simulink model "nonlinear_vs_linear"  (R2023a)
settings: Solver=ode1  StartTime=0.0  StopTime=200  FixedStep=1e-4  RelTol=1e-3
values from neighbouring files (symbols this model uses):
  alpha = 5    [comparison_of_two_C3s_for_positivity_issue.m]    (also in error_plots.m = 80; ns_vs_ls_sim.m = 80; output_response_gap_metrc_is_1.m = 80)
  beta = params(5)    [NS_parameter_generation.m]    (also in NS_parameter_generation_v2.m = params(4); comparison_of_two_C3s_for_positivity_issue.m = 75; error_plots.m = 75; ns_vs_ls_sim.m = 75)
  e3_0 = 2*(xr0 - x0(4))    [comparison_of_two_C3s_for_positivity_issue.m]    (also in error_plots.m; ns_vs_ls_sim.m; output_response_gap_metrc_is_1.m)
  eta = 75    [comparison_of_two_C3s_for_positivity_issue.m]    (also in error_plots.m; ns_vs_ls_sim.m; output_response_gap_metrc_is_1.m)
  K = 0.12    [comparison_of_two_C3s_for_positivity_issue.m]    (also in error_plots.m; ns_vs_ls_sim.m; output_response_gap_metrc_is_1.m)
  Ks = 0.15    [comparison_of_two_C3s_for_positivity_issue.m]    (also in error_plots.m; ns_vs_ls_sim.m; output_response_gap_metrc_is_1.m)
  Lambda = .08    (= 0.08)    [comparison_of_two_C3s_for_positivity_issue.m]    (also in error_plots.m; ns_vs_ls_sim.m; output_response_gap_metrc_is_1.m)
  x0 = [0;1e-8;0;500e-9]    [comparison_of_two_C3s_for_positivity_issue.m]    (also in error_plots.m; ns_vs_ls_sim.m = [5e-9;0e-5;0;500e-9]; output_response_gap_metrc_is_1.m = [5e-9;0;0;500e-9])
settings Model: Creator=guanyunliu  LastModifiedBy=guanyunliu

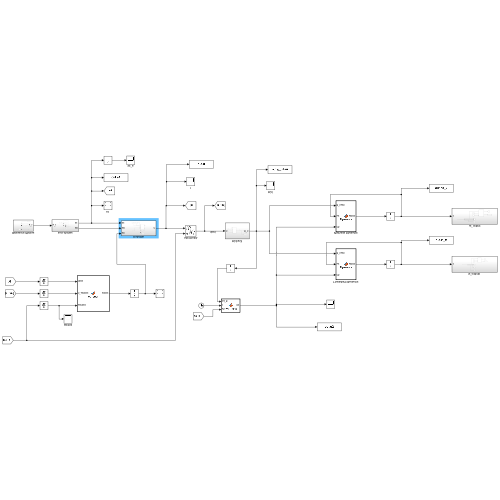
[thumbnail: Simulink's stored preview of the top-level diagram]
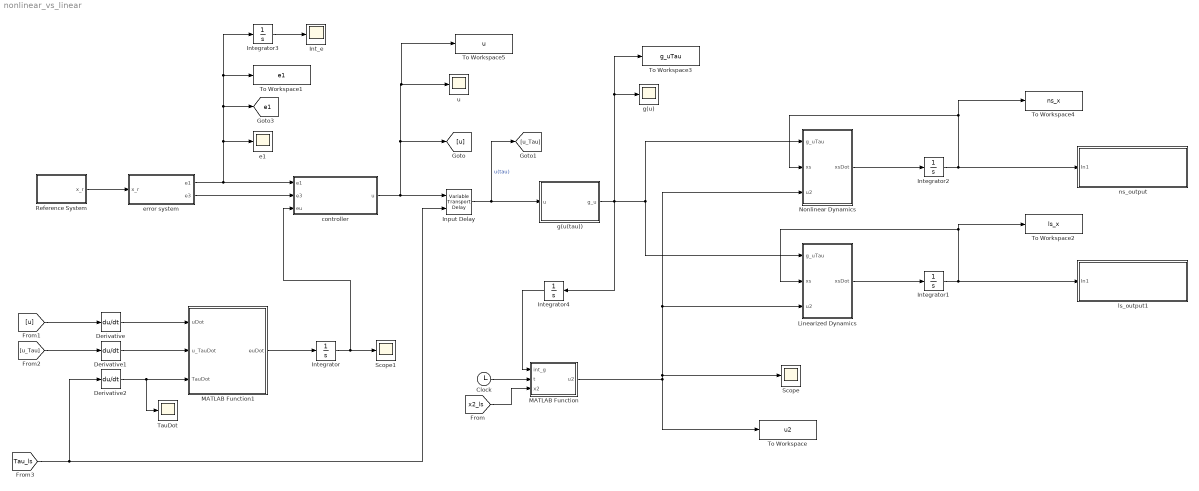
== system nonlinear_vs_linear ==
  Clock : Clock
  Derivative : Derivative
  Derivative1 : Derivative
  Derivative2 : Derivative
  Input Delay : VariableTransportDelay  VariableDelayType=Variable transport delay  MaximumDelay=10  MaximumPoints=100352
  Int_e : Scope
  Integrator : Integrator
  Integrator1 : Integrator  InitialCondition=x0
  Integrator2 : Integrator  InitialCondition=x0
  Integrator3 : Integrator
  Integrator4 : Integrator
  Linearized Dynamics : MATLAB Function  TreatAsAtomicUnit=on
  MATLAB Function : MATLAB Function  TreatAsAtomicUnit=on
  MATLAB Function1 : MATLAB Function  TreatAsAtomicUnit=on
  Nonlinear Dynamics : MATLAB Function  TreatAsAtomicUnit=on
  Reference System : Subsystem
  Scope : Scope
  Scope1 : Scope
  TauDot : Scope
  To Workspace : ToWorkspace  VariableName=u2  SaveFormat=Timeseries  SampleTime=-1
  To Workspace1 : ToWorkspace  VariableName=e1  SaveFormat=Timeseries  SampleTime=-1
  To Workspace2 : ToWorkspace  VariableName=ls_x  SaveFormat=Timeseries  SampleTime=-1
  To Workspace3 : ToWorkspace  VariableName=g_uTau  SaveFormat=Timeseries  SampleTime=-1
  To Workspace4 : ToWorkspace  VariableName=ns_x  SaveFormat=Timeseries  SampleTime=-1
  To Workspace5 : ToWorkspace  VariableName=u  SaveFormat=Timeseries  SampleTime=-1
  controller : Subsystem
  e1 : Scope
  error system : Subsystem
  g(u(tau)) : Subsystem
  g(u) : Scope
  ls_output1 : Subsystem
  ns_output : Subsystem
  u : Scope
  tag scope: e1=global
  wires:
  Reference System/1(x_r) -> error system/1(x_r)
  error system/1(e1) -> controller/1(e1), [e1], Integrator3/1, To Workspace1/1, e1/1
  error system/2(e3) -> controller/2(e3)
  controller/1(u) -> To Workspace5/1, u/1, [u], Input Delay/1
  Input Delay/1 -> [u_Tau], g(u(tau))/1(u)  "u(tau)"
  g(u(tau))/1(g_u) -> Integrator4/1, To Workspace3/1, g(u)/1, Nonlinear Dynamics/1(g_uTau), Linearized Dynamics/1(g_uTau)
  Nonlinear Dynamics/1(xsDot) -> Integrator2/1
  Linearized Dynamics/1(xsDot) -> Integrator1/1
  Integrator2/1 -> To Workspace4/1, Nonlinear Dynamics/2(xs), ns_output/1(In1)
  Integrator1/1 -> To Workspace2/1, Linearized Dynamics/2(xs), ls_output1/1(In1)
  [u_Tau] -> Derivative1/1
  MATLAB Function1/1(euDot) -> Integrator/1
  [u] -> Derivative/1
  Derivative/1 -> MATLAB Function1/1(uDot)
  Derivative1/1 -> MATLAB Function1/2(u_TauDot)
  Derivative2/1 -> TauDot/1, MATLAB Function1/3(TauDot)
  Integrator/1 -> Scope1/1, controller/3(eu)
  [Tau_ls] -> Derivative2/1, Input Delay/2
  MATLAB Function/1(u2) -> Scope/1, Nonlinear Dynamics/3(u2), Linearized Dynamics/3(u2), To Workspace/1
  Integrator3/1 -> Int_e/1
  Clock/1 -> MATLAB Function/2(t)
  Integrator4/1 -> MATLAB Function/1(int_g)
  [x2_ls] -> MATLAB Function/3(x2)

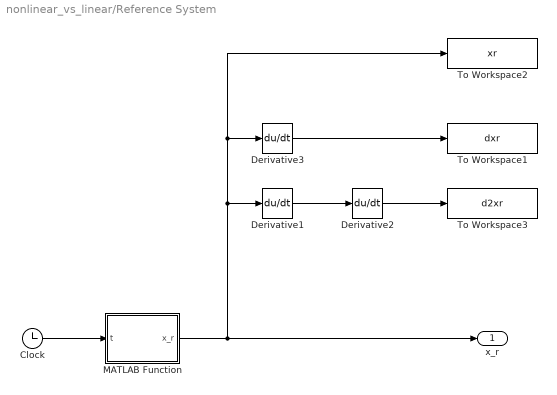
== system nonlinear_vs_linear/Reference System ==
  Clock : Clock
  Derivative1 : Derivative
  Derivative2 : Derivative
  Derivative3 : Derivative
  MATLAB Function : MATLAB Function  TreatAsAtomicUnit=on
  To Workspace1 : ToWorkspace  VariableName=dxr  SaveFormat=Timeseries  SampleTime=-1
  To Workspace2 : ToWorkspace  VariableName=xr  SaveFormat=Timeseries  SampleTime=-1
  To Workspace3 : ToWorkspace  VariableName=d2xr  SaveFormat=Timeseries  SampleTime=-1
  x_r : Outport
  wires:
  Clock/1 -> MATLAB Function/1(t)
  MATLAB Function/1(x_r) -> To Workspace2/1, Derivative3/1, Derivative1/1, x_r/1
  Derivative1/1 -> Derivative2/1
  Derivative2/1 -> To Workspace3/1
  Derivative3/1 -> To Workspace1/1

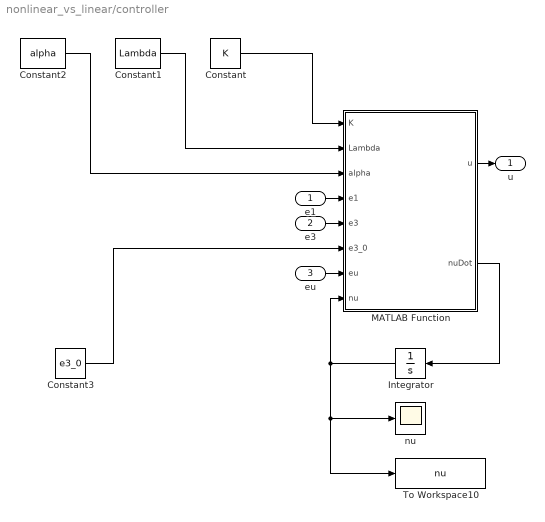
== system nonlinear_vs_linear/controller ==
  e1 : Inport
  e3 : Inport  Port=2
  eu : Inport  Port=3
  Constant : Constant  Value=K
  Constant1 : Constant  Value=Lambda
  Constant2 : Constant  Value=alpha
  Constant3 : Constant  Value=e3_0
  Integrator : Integrator
  MATLAB Function : MATLAB Function  TreatAsAtomicUnit=on
  To Workspace10 : ToWorkspace  VariableName=nu  SaveFormat=Timeseries  SampleTime=-1
  nu : Scope
  u : Outport
  wires:
  MATLAB Function/1(u) -> u/1
  e3/1 -> MATLAB Function/5(e3)
  Constant2/1 -> MATLAB Function/3(alpha)
  Constant/1 -> MATLAB Function/1(K)
  Constant3/1 -> MATLAB Function/6(e3_0)
  Constant1/1 -> MATLAB Function/2(Lambda)
  MATLAB Function/2(nuDot) -> Integrator/1
  e1/1 -> MATLAB Function/4(e1)
  Integrator/1 -> nu/1, To Workspace10/1, MATLAB Function/8(nu)
  eu/1 -> MATLAB Function/7(eu)

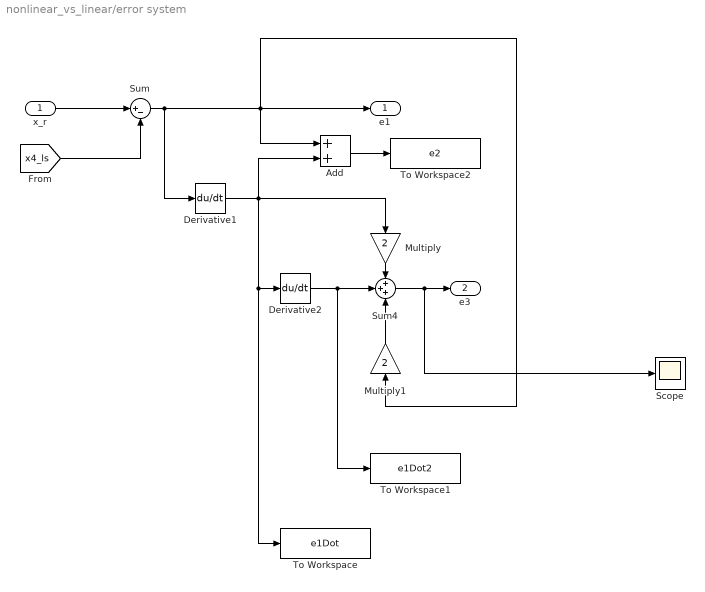
== system nonlinear_vs_linear/error system ==
  x_r : Inport
  Add : Sum
  Derivative1 : Derivative
  Derivative2 : Derivative
  Multiply : Gain  Gain=2
  Multiply1 : Gain  Gain=2
  Scope : Scope
  Sum : Sum  Inputs=|+-
  Sum4 : Sum  Inputs=+++
  To Workspace : ToWorkspace  VariableName=e1Dot  SaveFormat=Timeseries  SampleTime=-1
  To Workspace1 : ToWorkspace  VariableName=e1Dot2  SaveFormat=Timeseries  SampleTime=-1
  To Workspace2 : ToWorkspace  VariableName=e2  SaveFormat=Timeseries  SampleTime=-1
  e1 : Outport
  e3 : Outport  Port=2
  wires:
  x_r/1 -> Sum/1
  [x4_ls] -> Sum/2
  Sum/1 -> Derivative1/1, Add/1, e1/1, Multiply1/1
  Derivative2/1 -> To Workspace1/1, Sum4/2
  Multiply/1 -> Sum4/1
  Multiply1/1 -> Sum4/3
  Sum4/1 -> Scope/1, e3/1
  Derivative1/1 -> Add/2, Multiply/1, To Workspace/1, Derivative2/1
  Add/1 -> To Workspace2/1

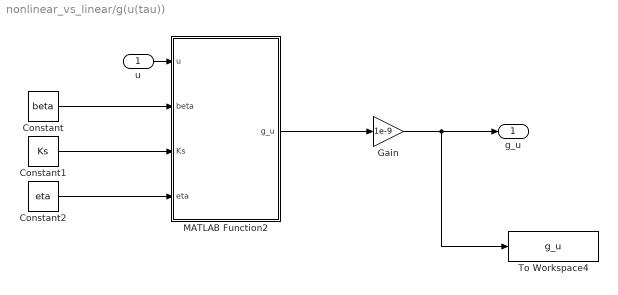
== system nonlinear_vs_linear/g(u(tau)) ==
  u : Inport
  Constant : Constant  Value=beta
  Constant1 : Constant  Value=Ks
  Constant2 : Constant  Value=eta
  Gain : Gain  Gain=1e-9
  MATLAB Function2 : MATLAB Function  TreatAsAtomicUnit=on
  To Workspace4 : ToWorkspace  VariableName=g_u  SaveFormat=Timeseries  SampleTime=-1
  g_u : Outport
  wires:
  Constant1/1 -> MATLAB Function2/3(Ks)
  Constant/1 -> MATLAB Function2/2(beta)
  u/1 -> MATLAB Function2/1(u)
  MATLAB Function2/1(g_u) -> Gain/1
  Constant2/1 -> MATLAB Function2/4(eta)
  Gain/1 -> To Workspace4/1, g_u/1

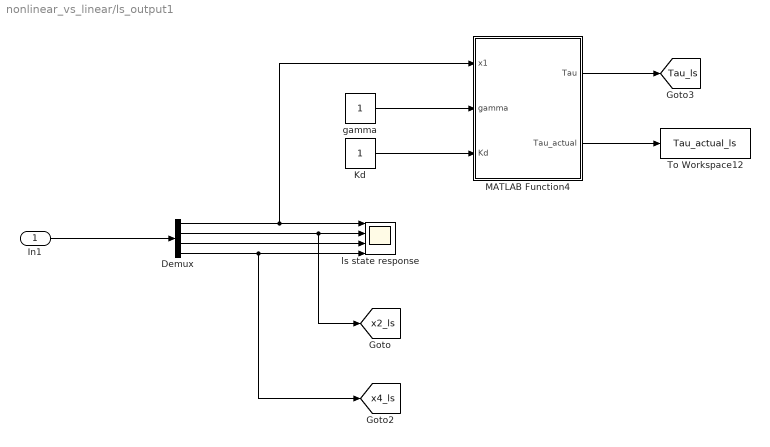
== system nonlinear_vs_linear/ls_output1 ==
  In1 : Inport
  Demux : Demux
  Kd : Constant
  MATLAB Function4 : MATLAB Function  TreatAsAtomicUnit=on
  To Workspace12 : ToWorkspace  VariableName=Tau_actual_ls  SaveFormat=Timeseries  SampleTime=-1
  gamma : Constant
  ls state response : Scope  NumInputPorts=4
  tag scope: Tau_ls=global, x2_ls=global, x4_ls=global
  wires:
  In1/1 -> Demux/1
  MATLAB Function4/2(Tau_actual) -> To Workspace12/1
  MATLAB Function4/1(Tau) -> [Tau_ls]
  Demux/1 -> MATLAB Function4/1(x1), ls state response/1
  Demux/4 -> [x4_ls], ls state response/4
  Kd/1 -> MATLAB Function4/3(Kd)
  gamma/1 -> MATLAB Function4/2(gamma)
  Demux/2 -> [x2_ls], ls state response/2
  Demux/3 -> ls state response/3

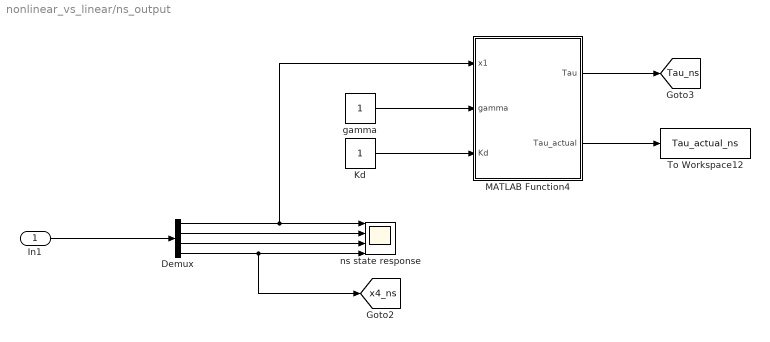
== system nonlinear_vs_linear/ns_output ==
  In1 : Inport
  Demux : Demux
  Kd : Constant
  MATLAB Function4 : MATLAB Function  TreatAsAtomicUnit=on
  To Workspace12 : ToWorkspace  VariableName=Tau_actual_ns  SaveFormat=Timeseries  SampleTime=-1
  gamma : Constant
  ns state response : Scope  NumInputPorts=4
  tag scope: Tau_ns=global, x4_ns=global
  wires:
  In1/1 -> Demux/1
  MATLAB Function4/2(Tau_actual) -> To Workspace12/1
  MATLAB Function4/1(Tau) -> [Tau_ns]
  Demux/1 -> MATLAB Function4/1(x1), ns state response/1
  Demux/4 -> [x4_ns], ns state response/4
  Kd/1 -> MATLAB Function4/3(Kd)
  gamma/1 -> MATLAB Function4/2(gamma)
  Demux/2 -> ns state response/2
  Demux/3 -> ns state response/3

== matlab function nonlinear_vs_linear/controller/MATLAB Function ==
  data: K input; u output; Lambda input; alpha input; e1 input; e3 input; e3_0 input; eu input; nu input; nuDot output
function [u, nuDot] = controller_u(K, Lambda, alpha, e1, e3, e3_0, eu, nu)
u = (sign(0.5 * (sign(e1) + 1))) * ...
    (K * (e3 - e3_0) + nu);
% if u <=0
%     u = 0;
% end
nuDot = K * (Lambda*e3+alpha*eu);
return

== matlab function nonlinear_vs_linear/Linearized Dynamics ==
  data: g_uTau input; xsDot output; xs input; u2 input; params parameter
function xsDot = Dynamics(g_uTau, xs, u2, params)
% xsDot = linearize_ode(xs, g_uTau, params);
xsDot = linearize_ode(xs, g_uTau, u2, params);

== matlab function nonlinear_vs_linear/g(u(tau))/MATLAB Function2 ==
  data: u input; g_u output; beta input; Ks input; eta input
function g_u = controller_g(u,beta, Ks, eta)

% g_u = ((beta/2)+((beta/2)*tanh(Ks/2*(u*1e9 - eta))))*1e-9;
g_u = ((beta/2)+((beta/2)*tanh(Ks/2*(u*1e9 - eta))));

return

== matlab function nonlinear_vs_linear/Nonlinear Dynamics ==
  data: g_uTau input; xsDot output; xs input; u2 input; params parameter
function xsDot = Dynamics(g_uTau, xs, u2, params)
% xsDot = nonlinear_ode(xs, g_uTau, params);
xsDot = nonlinear_ode(xs, g_uTau, u2, params);

== matlab function nonlinear_vs_linear/ns_output/MATLAB Function4 ==
  data: x1 input; Tau output; gamma input; Kd input; Tau_actual output
function [Tau, Tau_actual]= Delay(x1, gamma, Kd)
% Tau=(4.48*(max(x3,.202)^(-0.323))) ; From Damon's code
% Tau = gamma * x3^(-Kd);
Tau = gamma * 5^(-Kd);
Tau_actual = gamma * x1^(-Kd);
return

== matlab function nonlinear_vs_linear/ls_output1/MATLAB Function4 ==
  data: x1 input; Tau output; gamma input; Kd input; Tau_actual output
function [Tau, Tau_actual]= Delay(x1, gamma, Kd)
% Tau=(4.48*(max(x3,.202)^(-0.323))) ; From Damon's code
% Tau = gamma * x3^(-Kd);
% Tau = gamma * 5^(-Kd);
Tau = 0.2;
% Tau = 5;
if x1*1e3 <=0.1e-9
    Tau_actual = 10;
else 
    Tau_actual = gamma * (x1*1e3*1e9)^(-Kd);
end
% Tau = Tau_actual;
return

== matlab function nonlinear_vs_linear/MATLAB Function1 ==
  data: uDot input; euDot output; u_TauDot input; TauDot input
function euDot = eu_error(uDot,u_TauDot, TauDot)

euDot = -uDot+(1-TauDot)*u_TauDot;

== matlab function nonlinear_vs_linear/MATLAB Function ==
  data: int_g input; t input; x2 input; u2 output; params parameter
function u2 = FVII_Input(int_g, t, x2, params)
% u2 is calculated based on the magnitude of the ref signal at the steady
% state

% Regulation
% xr_ss = 130e-9;

% Sinusoidal Tracking
xr_ss = ref_signal(t);

% u2_trans = (-tanh(.2*t-2)+1)*0.5*params.beta*params.x20*int_g;
% u2_ss = (tanh(.2*t-2)+1)*0.5*(params.kd2*params.x20 + params.beta/params.gamma*params.kd3*params.kd4/params.kn4*xr_ss - params.kp2);
% u2 = u2_trans + u2_ss;
% u2=0;
% u2 = params.kd2*params.x20 + params.beta/params.gamma*params.kd3*params.kd4/params.kn4*xr_ss - params.kp2*(tanh(.2*t-2)+1)*0.5;
% u2 = 0;
u2 = params.kd2*params.x20 + params.beta/params.gamma*params.kd3*params.kd4/params.kn4*xr_ss;

% e2 = params.x20 - x2;
% u2 = params.beta*params.x20*int_g*sign(sign(e2)+1);

== matlab function nonlinear_vs_linear/Reference System/MATLAB Function ==
  data: t input; x_r output
function x_r = fcn(t)

x_r = ref_signal(t);
